simulink model "message_ros2_deserialize_receive_slrt"  (R2022b)
settings: Solver=FixedStepAuto  StartTime=0.0  StopTime=inf  RelTol=1e-3
libraries: ros2lib x1, simulink x1, ROSMessageSerializer x1, slrealtimeiplib x1
settings Model: Creator=jarisafi  LastModifiedBy=promero
settings SolverCC: ConcurrentTasks=on  AlgebraicLoopSolver=TrustRegion  PositivePriorityOrder=on  InsertRTBMode=Never (minimum delay)
settings DataIOCC: SaveFormat=StructureWithTime  ReturnWorkspaceOutputs=off
settings OptimizationCC: BlockReduction=off  OptimizeBlockIOStorage=off  BufferReuse=off  GlobalBufferReuse=off  ExpressionFolding=off  LocalBlockOutputs=off
settings DebuggingCC: TasksWithSamePriorityMsg=none  UnconnectedInputMsg=warning  UnconnectedOutputMsg=warning  UnconnectedLineMsg=warning  SFMachineParentedDataDiag=warning  ArithmeticOperatorsInVariantConditions=warning
settings HardwareCC: ProdBitPerLong=64  ProdLongLongMode=on  ProdHWDeviceType=Intel->x86-64 (Linux 64)
settings ModelReferenceCC: EnableRefExpFcnMdlSchedulingChecks=on
settings SFSimCC: SimUseLocalCustomCode=off  CustomCodeUndefinedFunction=UseInterfaceOnly
settings RTWCC: Description=Simulink Real-Time  SystemTargetFile=slrealtime.tlc  PackageName=packNgo_out.zip  TemplateMakefile=slrealtime_default_tmf  RTWUseLocalCustomCode=off  Toolchain=Simulink Real-Time Toolchain  BuildConfiguration=Faster Runs  CodeExecutionProfiling=on  TargetLang=C++  DLArmComputeVersion=19.05
settings CodeAppCC: StateflowObjectComments=on

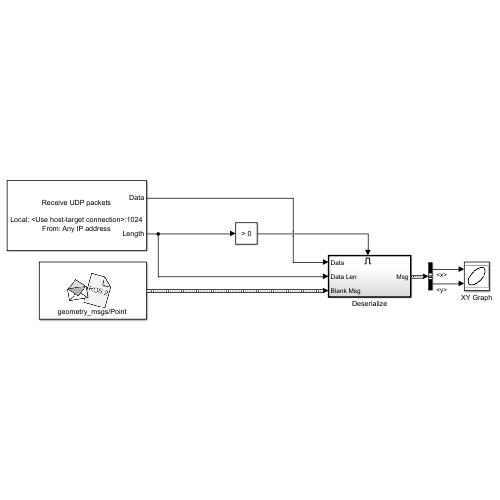
[thumbnail: Simulink's stored preview of the top-level diagram]
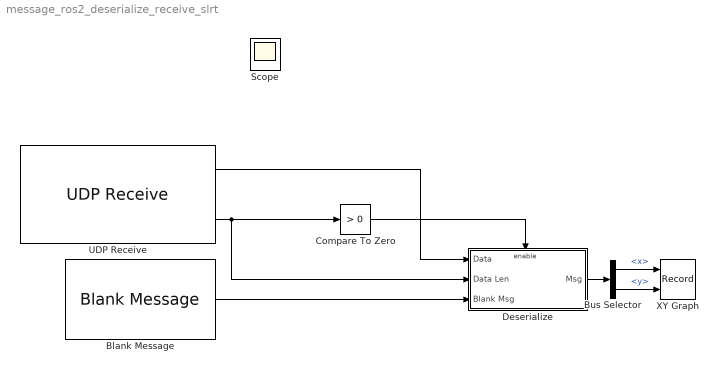
== system message_ros2_deserialize_receive_slrt ==
  Blank Message : ros2lib/Blank Message  messageClass=Message  entityType=geometry_msgs/Point  messageType=geometry_msgs/Point  SampleTime=inf
  Bus Selector : BusSelector  OutputSignals=x,y
  Compare To Zero : simulink/Logic and Bit Operations/Compare To Zero  relop=>  OutDataTypeStr=boolean
  Deserialize : Subsystem  TreatAsAtomicUnit=on
  UDP Receive : slrealtimeiplib/UDP Receive  useHostTargetConn=on  ipAddress=10.10.10.15  localPort=1024  rcvWidth=16  rcvFmAny=on  fmAddress='10.10.10.10'  sampleTime=0.05  enableMessage=off  maxPackets=1
  XY Graph : Record  FileSettingsInternal="{\"entries\":[{\"content\":{\"excelSettings\":{\"content\":{},\"type\":\"Streamout.ExcelSettings\"}},\"type\":\"Streamout.FileSettingStorage\",\"uuid\":\"20c77975-f111-44cf-a182-5aae3217dd01\"}],\"packageUris\":[\"http://schema.mathworks.com/mf0/streamout_blocks/R2020a\"],\"version\":\"1.0\"}"  Layout=[1 1]  SignalsInternal="{\"entries\":[{\"content\":{\"signals\":[{\"content\":{\"blockPath\":[\"message_ros2_deserialize_receive_slrt/XY Graph\"],\"channel\":[],\"dimensions\":[1],\"domain\":\"message_ros2_deserialize_receive_slrt/XY Graph\",\"lineColor\":\"#a2142f\",\"plots\":[1],\"port\":1,\"sid\":[],\"signalID\":1126,\"signalName\":\"XY Graph:1\"},\"type\":\"RecordBlkView.Signal\",\"uuid\":\"4b7c1e82-1e3c-4519-9b8b-d933062b77dd\"},{\"content\":{\"blockPath\":[\"message_ros2_deserialize_receive_slrt/XY Graph\"],\"channel\":[],\"dimensions\":[1],\"domain\":\"message_ros2_deserialize_receive_slrt/XY Graph\",\"lineColor\":\"#139fff\",\"plots\":[1],\"port\":2,\"sid\":[],\"signalID\":1129,\"signalName\":\"XY Graph:2\"},\"type\":\"RecordBlkView.Signal\",\"uuid\":\"273f5fd4-4b02-49d0-b680-bf0cb2a6d827\"}]},\"type\":\"RecordBlkView.InputSignals\",\"uuid\":\"b40b3820-72a2-4892-99bc-309cbd14564e\"}],\"packageUris\":[\"http://schema.mathworks.com/mf0/streamout_blocks/R2020a\"],\"version\":\"1.0\"}"  VisualizationBindings="{\"xyplotplugin\":{\"info\":[{\"series\":[{\"bindingParametersList\":[{\"parameter\":\"X-Axis\",\"signalID\":1126,\"signalName\":\"XY Graph:1\"},{\"parameter\":\"Y-Axis\",\"signalID\":1129,\"signalName\":\"XY Graph:2\"}],\"seriesID\":13810}],\"subplotID\":1}]}}"  CompatibilityTag=XY  st=-1
  Scope : Scope
  wires:
  Blank Message/1 -> Deserialize/3(Blank Msg)
  UDP Receive/2 -> Compare To Zero/1, Deserialize/2(Data Len)
  UDP Receive/1 -> Deserialize/1(Data)
  Deserialize/1(Msg) -> Bus Selector/1
  Bus Selector/1 -> XY Graph/1  "<x>"
  Bus Selector/2 -> XY Graph/2  "<y>"
  Compare To Zero/1 -> Deserialize/Enable

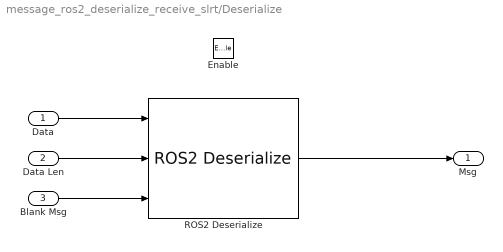
== system message_ros2_deserialize_receive_slrt/Deserialize ==
  Data : Inport
  Data Len : Inport  Port=2
  Blank Msg : Inport  Port=3
  Enable : EnablePort  PropagateVarSize=During execution
  ROS2 Deserialize : ROSMessageSerializer/ROS2 Deserialize  MessageType=geometry_msgs/Point  SimulateUsing=Code generation
  Msg : Outport
  wires:
  Data/1 -> ROS2 Deserialize/1
  ROS2 Deserialize/1 -> Msg/1
  Data Len/1 -> ROS2 Deserialize/2
  Blank Msg/1 -> ROS2 Deserialize/3
